simulink model "LED - Simulink scheme"  (R2020b)
settings: Solver=VariableStepAuto  StartTime=0.0  StopTime=10.0  MaxStep=1e-6  RelTol=1e-9
libraries: nesl_utility x28, fl_lib x22, ee_lib x20, simulink x4
settings Model: Creator=claudio.rossi  LastModifiedBy=Gioele
settings SolverCC: ZeroCrossAlgorithm=Adaptive
settings DebuggingCC: IgnoredZcDiagnostic=none
settings SFSimCC: CustomCodeUndefinedFunction=UseInterfaceOnly

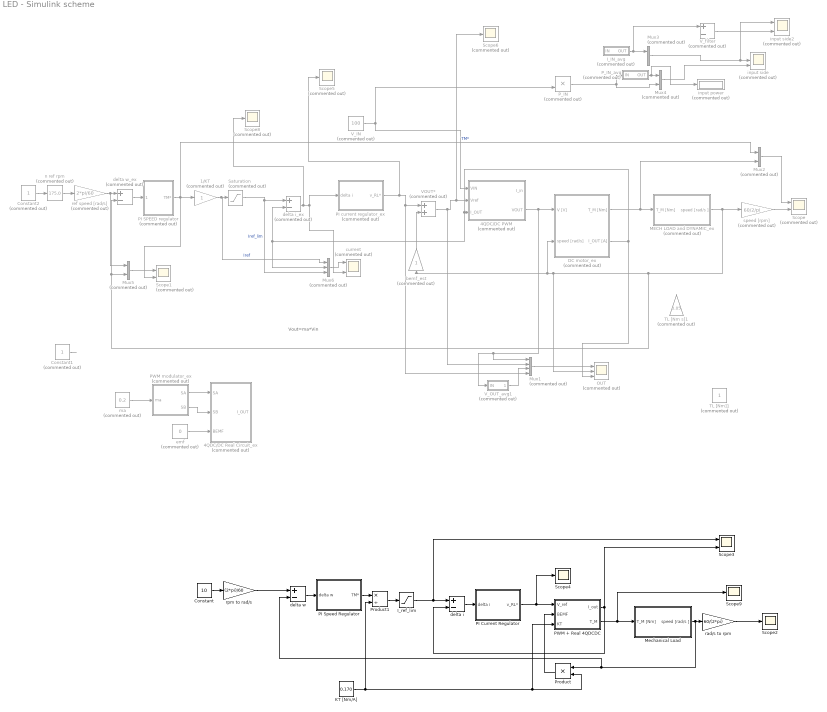
== system LED - Simulink scheme ==
  note: Vout=ma*Vin
  1/KT : Gain  Commented=on
  4QDC/DC PWM : Subsystem  Commented=on
  4QDC/DC Real Circuit_ex : Subsystem  Commented=on
  Constant : Constant  Value=10
  Constant1 : Constant  Commented=on
  Constant2 : Constant  Commented=on
  DC motor_ex : Subsystem  Commented=on
  I_IN_avg : Subsystem  Commented=on  mask{Ts=0.001}
      mask prompts: Ts "period [s]"
  I_ref_lim : Saturate  UpperLimit=1.8  LowerLimit=-1.7
  KT [Nm/A] : Constant  Value=0.170
  MECH LOAD and DYNAMIC_ex : Subsystem  Commented=on
  Mechanical Load : Subsystem
  Mux1 : Mux  Commented=on
  Mux{2..5} (4 alike) : Mux  Commented=on  Inputs=2
  Mux6 : Mux  Commented=on  Inputs=3
  OUT : Scope  Commented=on  NumInputPorts=3
  PI Current Regulator : Subsystem
  PI SPEED regulator : Subsystem  Commented=on
  PI Speed Regulator : Subsystem
  PI current regulator_ex : Subsystem  Commented=on
  "PWM + Real 4QDCDC " : Subsystem
  PWM modulator_ex : Subsystem  Commented=on
  P_IN : Product  Commented=on
  P_IN_avg : Subsystem  Commented=on  mask{Ts=0.001}
      mask prompts: Ts "period [s]"
  Product : Product
  Product1 : Product  Inputs=*/
  Saturation : Saturate  Commented=on  UpperLimit=5  LowerLimit=-5
  Scope : Scope  Commented=on  NumInputPorts=2
  Scope1 : Scope  Commented=on  NumInputPorts=2
  Scope2 : Scope
  Scope3 : Scope  NumInputPorts=2
  Scope4 : Scope
  Scope5 : Scope  Commented=on
  Scope6 : Scope  Commented=on
  Scope8 : Scope  Commented=on
  Scope9 : Scope
  TL [Nm s]1 : Gain  Commented=on  Gain=0.05
  TL [Nm]1 : Constant  Commented=on
  VOUT* : Sum  Commented=on
  V_IN : Constant  Commented=on  Value=100
  V_OUT_avg1 : Subsystem  Commented=on  mask{Ts=0.00005}
      mask prompts: Ts "period"
  V_filter : Sum  Commented=on  Inputs=+-
  bemf_est : Gain  Commented=on
  current : Scope  Commented=on  NumInputPorts=2
  delta i : Sum  Inputs=+-
  delta i_ex : Sum  Commented=on  Inputs=+-
  delta w : Sum  Inputs=+-
  delta w_ex : Sum  Commented=on  Inputs=+-
  emf : Constant  Commented=on  Value=0
  input power : Display  Commented=on
  input side : Scope  Commented=on  NumInputPorts=3
  input side2 : Scope  Commented=on  NumInputPorts=2
  ma : Constant  Commented=on  Value=0.2
  n ref rpm : simulink/Math Operations/Slider Gain  Commented=on  gain=175.0  low=-500  high=1000
  rad/s to rpm : Gain  Gain=60/(2*pi)
  ref speed [rad/s] : Gain  Commented=on  Gain=2*pi/60
  rpm to rad/s : Gain  Gain=(2*pi)/60
  speed [rpm] : Gain  Commented=on  Gain=60/2/pi
  wires:
  ma/1 -> PWM modulator_ex/1(ma)
  PWM modulator_ex/1(SA) -> 4QDC/DC Real Circuit_ex/1(SA)
  PWM modulator_ex/2(SB) -> 4QDC/DC Real Circuit_ex/2(SB)
  emf/1 -> 4QDC/DC Real Circuit_ex/3(BEMF)
  Constant1/1 -> ?
  Saturation/1 -> Mux6/3, delta i_ex/1  "Iref_lim"
  Mux3/1 -> input side2/1, input side/2
  ref speed [rad/s]/1 -> Mux5/1, delta w_ex/1
  Mux5/1 -> Scope1/1
  Constant2/1 -> n ref rpm/1
  delta w_ex/1 -> PI SPEED regulator/1(delta w)
  n ref rpm/1 -> ref speed [rad/s]/1
  speed [rpm]/1 -> Scope/2
  PI SPEED regulator/1(TM*) -> 1/KT/1, Mux2/1, Scope1/2  "TM*"
  DC motor_ex/1(T_M [Nm]) -> Mux2/2, MECH LOAD and DYNAMIC_ex/1(T_M [Nm])
  Mux4/1 -> input side/3
  V_IN/1 -> 4QDC/DC PWM/1(VIN), P_IN/2
  Mux2/1 -> Scope/1
  MECH LOAD and DYNAMIC_ex/1(speed [rad/s ]) -> Mux5/2, delta w_ex/2, OUT/2, bemf_est/1, DC motor_ex/2(speed [rad/s]), speed [rpm]/1
  I_IN_avg/1(OUT) -> V_filter/1, Mux3/1
  Mux6/1 -> current/1
  4QDC/DC PWM/2(VOUT) -> V_OUT_avg1/1(IN), Mux1/1, DC motor_ex/1(V [V])
  PI current regulator_ex/1(v_RL*) -> Scope5/1, Mux1/4, VOUT*/1
  DC motor_ex/2(I_OUT [A]) -> OUT/3, delta i_ex/2, Mux6/2, 4QDC/DC PWM/3(I_OUT)
  V_OUT_avg1/1(OUT) -> Mux1/3
  delta i_ex/1 -> Scope8/1, PI current regulator_ex/1(delta i), current/2
  1/KT/1 -> Mux6/1, Saturation/1  "Iref"
  VOUT*/1 -> Mux1/2, Scope6/1, 4QDC/DC PWM/2(Vref)
  bemf_est/1 -> VOUT*/2
  P_IN/1 -> Mux4/2, P_IN_avg/1(IN)
  P_IN_avg/1(OUT) -> input power/1, Mux4/1
  Mux1/1 -> OUT/1
  V_filter/1 -> input side2/2
  Product/1 -> "PWM + Real 4QDCDC "/2(BEMF)
  "PWM + Real 4QDCDC "/2(T_M) -> Scope9/1, Mechanical Load/1(T_M [Nm])
  KT [Nm/A]/1 -> Product/2, "PWM + Real 4QDCDC "/3(KT), Product1/2
  PI Current Regulator/1(v_RL*) -> Scope4/1, "PWM + Real 4QDCDC "/1(V_ref)
  delta i/1 -> PI Current Regulator/1(delta i)
  Product1/1 -> I_ref_lim/1
  PI Speed Regulator/1(TM*) -> Product1/1
  delta w/1 -> PI Speed Regulator/1(delta w)
  rad/s to rpm/1 -> Scope2/1
  rpm to rad/s/1 -> delta w/1
  Constant/1 -> rpm to rad/s/1
  I_ref_lim/1 -> delta i/1, Scope3/1
  Mechanical Load/1(speed [rad/s ]) -> delta w/2, Product/1, rad/s to rpm/1
  "PWM + Real 4QDCDC "/1(I_out) -> Scope3/2, delta i/2

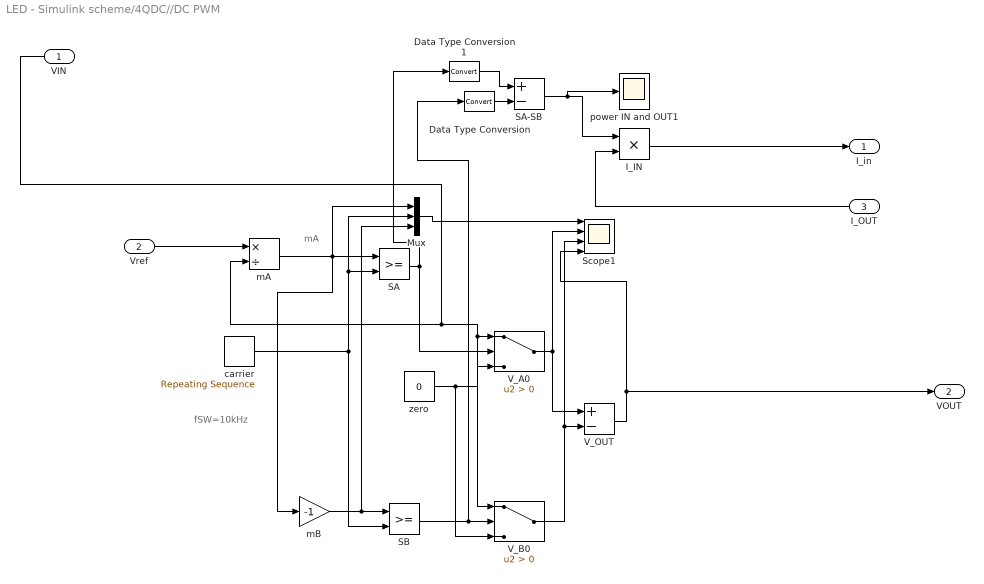
== system LED - Simulink scheme/4QDC//DC PWM ==
  note: mA
  note: fSW=10kHz
  VIN : Inport
  Vref : Inport  Port=2
  I_OUT : Inport  Port=3
  Data Type Conversion : DataTypeConversion
  Data Type Conversion1 : DataTypeConversion
  I_IN : Product
  Mux : Mux  Inputs=3
  SA : RelationalOperator  OutDataTypeStr=boolean  RndMeth=Simplest
  SA-SB : Sum  Inputs=+-
  SB : RelationalOperator  OutDataTypeStr=boolean  RndMeth=Simplest
  Scope1 : Scope  NumInputPorts=4
  V_A0 : Switch  Criteria=u2 > Threshold
  V_B0 : Switch  Criteria=u2 > Threshold
  V_OUT : Sum  Inputs=+-
  carrier : simulink/Sources/Repeating Sequence  rep_seq_t=[0 1e-4/2 1e-4]  rep_seq_y=[-1 1 -1]
  mA : Product  Inputs=*/
  mB : Gain  Gain=-1
  power IN and OUT1 : Scope
  zero : Constant  Value=0
  I_in : Outport  VectorParamsAs1DForOutWhenUnconnected=off
  VOUT : Outport  Port=2  VectorParamsAs1DForOutWhenUnconnected=off
  wires:
  I_IN/1 -> I_in/1
  zero/1 -> V_B0/3, V_A0/3
  carrier/1 -> SB/2, Mux/2, SA/2
  Mux/1 -> Scope1/1
  mA/1 -> mB/1, Mux/1, SA/1
  V_A0/1 -> Scope1/2, V_OUT/1
  VIN/1 -> V_B0/1, V_A0/1, mA/2
  V_OUT/1 -> Scope1/4, VOUT/1
  SA/1 -> Data Type Conversion1/1, V_A0/2
  I_OUT/1 -> I_IN/2
  SB/1 -> Data Type Conversion/1, V_B0/2
  V_B0/1 -> Scope1/3, V_OUT/2
  Data Type Conversion/1 -> SA-SB/2
  SA-SB/1 -> power IN and OUT1/1, I_IN/1
  mB/1 -> SB/1, Mux/3
  Data Type Conversion1/1 -> SA-SB/1
  Vref/1 -> mA/1

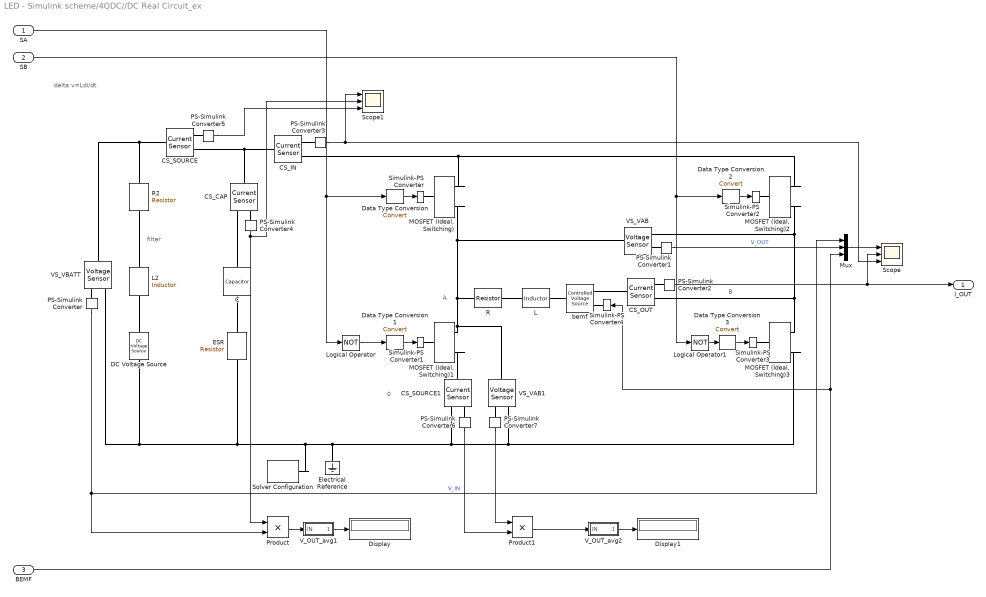
== system LED - Simulink scheme/4QDC//DC Real Circuit_ex ==
  note: filter
  note: B
  note: 0
  note: A
  note: delta v=Ldi/dt
  SA : Inport
  SB : Inport  Port=2
  BEMF : Inport  Port=3
  C : ee_lib/Passive/Capacitor  cap_option=0  c=1e-3 F  Cvec=[1e-05, 1e-06] F  Vvec=[0, 10] V  CV_table_symmetry=1  f_vec=[1, 10] kHz  DFext_vec=[.8, 1.2]  C_tol=5  enable_C_tol=0  tol_distribution=1  nSigma=4  r=1e-6 Ohm  g=0 1/Ohm  averaging_period=0 s  enable_operating_limits=0  operating_limit_action=2  max_working_voltage_range=[-25, 25] V  power_rating=1 W  enable_faults=0  fault_action=1  Cscale_faulted=100  R_faulted=1e-3 Ohm  G_faulted=0 1/Ohm  tau_fault=1e-3 s  enable_temporal_fault=0  t_fault=1 s  enable_behavioral_fault=0  max_permissible_voltage_range=[-100, 100] V  t_fail_on_voltage=1 s  i_specify=off  i_priority=None  i=0 A  i_nominal_specify=off  i_nominal_unit=A  i_nominal_value=1  v_specify=off  v_priority=None  v=0 V  v_nominal_specify=off  v_nominal_unit=V  v_nominal_value=1  vc_specify=off  vc_priority=High  vc=0 V  vc_nominal_specify=off  vc_nominal_unit=V  vc_nominal_value=1
  CS_CAP : fl_lib/Electrical/Electrical Sensors/Current Sensor
  CS_IN : fl_lib/Electrical/Electrical Sensors/Current Sensor
  CS_OUT : fl_lib/Electrical/Electrical Sensors/Current Sensor
  CS_SOURCE : fl_lib/Electrical/Electrical Sensors/Current Sensor
  CS_SOURCE1 : fl_lib/Electrical/Electrical Sensors/Current Sensor
  DC Voltage Source : fl_lib/Electrical/Electrical Sources/DC Voltage Source  v0=100 V
  Data Type Conversion{,1..3} (4 alike) : DataTypeConversion
  Display : Display
  Display1 : Display
  ESR : ee_lib/Passive/Resistor  R=0.01 Ohm  R_tol=5  enable_R_tol=0  tol_distribution=1  nSigma=4  enable_operating_limits=0  operating_limit_action=2  max_working_voltage=100 V  power_rating=1 W  enable_faults=0  fault_action=1  R_faulted=inf Ohm  enable_temporal_fault=0  t_fault=1 s  enable_behavioral_fault=0  max_permissible_current=1 A  t_fail_on_current=1 s  noise_mode=0  sample_time=1e-3 s  repeatability=1  auto_seed=249578223  user_seed=0  Tdevice=25 degC  alpha=3.93e-3 1/K  Tmeas=25 degC  thermal_mass=100 J/K  power_derating_T1=70 degC  power_derating_T2=155 degC  operating_temperature_range_vec=[-50, 150] degC  temperature_specify=off  temperature_priority=High  temperature=298.15 K  temperature_nominal_specify=off  temperature_nominal_unit=K  temperature_nominal_value=1
  Electrical Reference : fl_lib/Electrical/Electrical Elements/Electrical Reference
  L : ee_lib/Passive/Inductor  l=10e-3 H  L_tol=20  enable_L_tol=0  tol_distribution=1  nSigma=4  r=0 Ohm  g=1e-9 1/Ohm  enable_operating_limits=0  operating_limit_action=2  max_working_current=1 A  power_rating=1 W  enable_faults=0  fault_action=1  lambdaPercent=50  k_faulted=0.9999  turnsShort=0  openCct=0  groundShort=0  groundShortG=0 1/Ohm  tau_fault=1e-3 s  enable_temporal_fault=0  t_fault=1 s  enable_behavioral_fault=0  max_permissible_voltage=100 V  n_fail_on_voltage=1  max_permissible_current=1 A  t_fail_on_current=1 s  i_L_specify=off  i_L_priority=High  i_L=0 A  i_L_nominal_specify=off  i_L_nominal_unit=A  i_L_nominal_value=1
  L2 : ee_lib/Passive/Inductor  l=1e-5 H  L_tol=20  enable_L_tol=0  tol_distribution=1  nSigma=4  r=0 Ohm  g=1e-9 1/Ohm  enable_operating_limits=0  operating_limit_action=2  max_working_current=1 A  power_rating=1 W  enable_faults=0  fault_action=1  lambdaPercent=50  k_faulted=0.9999  turnsShort=0  openCct=0  groundShort=0  groundShortG=0 1/Ohm  tau_fault=1e-3 s  enable_temporal_fault=0  t_fault=1 s  enable_behavioral_fault=0  max_permissible_voltage=100 V  n_fail_on_voltage=1  max_permissible_current=1 A  t_fail_on_current=1 s  i_L_specify=off  i_L_priority=High  i_L=0 A  i_L_nominal_specify=off  i_L_nominal_unit=A  i_L_nominal_value=1
  Logical Operator : Logic  Operator=NOT  AllPortsSameDT=off  OutDataTypeStr=boolean
  Logical Operator1 : Logic  Operator=NOT  AllPortsSameDT=off  OutDataTypeStr=boolean
  MOSFET (Ideal, Switching){,1..3} (4 alike) : ee_lib/Semiconductors & Converters/MOSFET (Ideal, Switching)  Rds=0.1 Ohm  Goff=1e-6 1/Ohm  Vth=0.5 V  diode_param=1  diode_Vf=0.8 V  diode_Ron=0.001 Ohm  diode_Goff=1e-5 1/Ohm  diode_C=50e-9 F  diode_iRM=-235 A  diode_iF=300 A  diode_idot=-50 A/us  diode_trr_param=1  diode_trr_factor=3  diode_trr=15 us  diode_Qrr=1500 s*uA  thermal_loss_option=2  Von_data=[0, 1.1, 1.3, 1.45, 1.75, 2.25, 2.7; 0, 1, 1.15, 1.35, 1.7, 2.35, 3] V  Eon_data=[0, .29, 1.43, 2.86, 5.71, 13.14, 22.86; 0, .57, 2.63, 5.14, 10.29, 20.57, 30.29] * 1e-3 J  Eoff_data=[0, .21, 1.07, 2.14, 4.29, 9.86, 17.14; 0, .43, 1.97, 3.86, 7.71, 15.43, 22.71] * 1e-3 J  Tj=[298.15, 398.15] K  Iout_data=[0, 10, 50, 100, 200, 400, 600] A  Eon_scalar=22.86e-3 J  Eoff_scalar=17.14e-3 J  Voff=300 V  Iout_scalar=600 A  diodeModelType=ee.enum.converters.diodeModelType.pwl  diode_IfMat=[.07, .12, .19, 1.75, 4.24, 7.32, 11.2; .16, .3, .72, 2.14, 4.02, 6.35, 9.12] A  diode_TjVec=[25, 125] degC  diode_VfVec=[.5, .7, .9, 1.3, 1.7, 2.1, 2.5] V  thermal_network_parameterization=ee.enum.thermalNetworkTopology.external  Rth=[.03, .2] K/W  Rth_Foster=[.03, .2] K/W  thermal_mass_parameterization=ee.enum.thermalNetwork.timeconstant  thermal_mass=[3, 25] J/K  thermal_mass_Foster=[33, 50] J/K  thermal_time_constant=[.1, 5] s  thermal_time_constant_Foster=[1, 10] s  thermal_mass_initial_temperatures=[25, 25] degC  junction_thermal_mass=0.1 J/K  Tau=1e-4 s  vT_specify=off  vT_priority=None  vT=0 V  vT_nominal_specify=off  vT_nominal_unit=V  vT_nominal_value=1  Qj_specify=off  Qj_priority=None  Qj=0 W  Qj_nominal_specify=off  Qj_nominal_unit=W  Qj_nominal_value=1  junction_temperature_specify=off  junction_temperature_priority=None  junction_temperature=25 degC  junction_temperature_nominal_specify=off  junction_temperature_nominal_unit=degC  junction_temperature_nominal_value=1
  Mux : Mux  Inputs=3
  PS-Simulink Converter{,1..7} (8 alike) : nesl_utility/PS-Simulink Converter  PhysicalDomain=network_engine_domain  SubClassName=ps_output  LeftPortType=input  RightPortType=output  PseudoPeriodic=off  Frequencies=[]  Unit=1  AffineConversion=off
  Product : Product
  Product1 : Product
  R : ee_lib/Passive/Resistor  R=10 Ohm  R_tol=5  enable_R_tol=0  tol_distribution=1  nSigma=4  enable_operating_limits=0  operating_limit_action=2  max_working_voltage=100 V  power_rating=1 W  enable_faults=0  fault_action=1  R_faulted=inf Ohm  enable_temporal_fault=0  t_fault=1 s  enable_behavioral_fault=0  max_permissible_current=1 A  t_fail_on_current=1 s  noise_mode=0  sample_time=1e-3 s  repeatability=1  auto_seed=1734551367  user_seed=0  Tdevice=25 degC  alpha=3.93e-3 1/K  Tmeas=25 degC  thermal_mass=100 J/K  power_derating_T1=70 degC  power_derating_T2=155 degC  operating_temperature_range_vec=[-50, 150] degC  temperature_specify=off  temperature_priority=High  temperature=298.15 K  temperature_nominal_specify=off  temperature_nominal_unit=K  temperature_nominal_value=1
  R2 : ee_lib/Passive/Resistor  R=0.1 Ohm  R_tol=5  enable_R_tol=0  tol_distribution=1  nSigma=4  enable_operating_limits=0  operating_limit_action=2  max_working_voltage=100 V  power_rating=1 W  enable_faults=0  fault_action=1  R_faulted=inf Ohm  enable_temporal_fault=0  t_fault=1 s  enable_behavioral_fault=0  max_permissible_current=1 A  t_fail_on_current=1 s  noise_mode=0  sample_time=1e-3 s  repeatability=1  auto_seed=3714298798  user_seed=0  Tdevice=25 degC  alpha=3.93e-3 1/K  Tmeas=25 degC  thermal_mass=100 J/K  power_derating_T1=70 degC  power_derating_T2=155 degC  operating_temperature_range_vec=[-50, 150] degC  temperature_specify=off  temperature_priority=High  temperature=298.15 K  temperature_nominal_specify=off  temperature_nominal_unit=K  temperature_nominal_value=1
  Scope : Scope  NumInputPorts=3
  Scope1 : Scope  NumInputPorts=3
  Simulink-PS Converter{,1..4} (5 alike) : nesl_utility/Simulink-PS Converter  PhysicalDomain=network_engine_domain  SubClassName=ps_input  LeftPortType=input  RightPortType=output  PseudoPeriodic=off  Frequencies=[]  NoiseDistribution=none  NoiseParameters=[]  Unit=1  AffineConversion=off  FilteringAndDerivatives=provide  SimscapeFilterOrder=1  InputFilterTimeConstant=0.001  UdotUserProvided=0
  Solver Configuration : nesl_utility/Solver Configuration  PhysicalDomain=network_engine_domain  SubClassName=solver  LeftPortType=input  RightPortType=generic  Tones=[]  Harmonics=[]  SimulateNoise=off  Profile=off  UseLocalSampling=off  EnableSwitchedLinearOptims=on  FrequencyDomain=off  UseCCode=off  RelTol=0.001  AbsTol=1e-06  MinStep=1e-09  ToWorkspace=off  RevertToSquareIcSolve=off  NumHomotopyIterations=100  PhasorMode=off  PhasorModeNumHarmonics=1  DoDC=off  ResidualTolerance=1e-09  UseLocalSolver=off  LocalSolverChoice=NE_BACKWARD_EULER_ADVANCER  LocalSolverSampleTime=0.001  DoFixedCost=off  MaxNonlinIter=3  MaxModeIter=2  ComputeImpulses=off  ImpulseIterations=2  LinearAlgebra=auto  EquationFormulation=NE_TIME_EF  DelaysMemoryBudget=1024  AutomaticFiltering=on  FilteringTimeConstant=0.001  PartitionStorageMethod=AS_NEEDED  PartitionMemoryBudget=1024  PartitionMethod=ROBUST
  VS_VAB : fl_lib/Electrical/Electrical Sensors/Voltage Sensor
  VS_VAB1 : fl_lib/Electrical/Electrical Sensors/Voltage Sensor
  VS_VBATT : fl_lib/Electrical/Electrical Sensors/Voltage Sensor
  V_OUT_avg1 : Subsystem  mask{Ts=0.0001}
      mask prompts: Ts "period"
  V_OUT_avg2 : Subsystem  mask{Ts=0.0001}
      mask prompts: Ts "period"
  bemf : fl_lib/Electrical/Electrical Sources/Controlled Voltage Source
  I_OUT : Outport  VectorParamsAs1DForOutWhenUnconnected=off
  wires:
  BEMF/1 -> Simulink-PS Converter4/1, Mux/3
  PS-Simulink Converter2/1 -> Scope/2, I_OUT/1
  PS-Simulink Converter3/1 -> Scope1/1, Scope/3
  Logical Operator/1 -> Data Type Conversion1/1
  SA/1 -> Data Type Conversion/1, Logical Operator/1
  Mux/1 -> Scope/1
  Data Type Conversion/1 -> Simulink-PS Converter/1
  Data Type Conversion1/1 -> Simulink-PS Converter1/1
  PS-Simulink Converter/1 -> Product/2, Mux/1  "V_IN"
  PS-Simulink Converter1/1 -> Mux/2  "V_OUT"
  Data Type Conversion2/1 -> Simulink-PS Converter2/1
  PS-Simulink Converter4/1 -> Product/1, Scope1/2
  PS-Simulink Converter5/1 -> Scope1/3
  Product/1 -> V_OUT_avg1/1(IN)
  V_OUT_avg1/1(OUT) -> Display/1
  PS-Simulink Converter7/1 -> Product1/1
  PS-Simulink Converter6/1 -> Product1/2
  Product1/1 -> V_OUT_avg2/1(IN)
  V_OUT_avg2/1(OUT) -> Display1/1
  Data Type Conversion3/1 -> Simulink-PS Converter3/1
  SB/1 -> Logical Operator1/1, Data Type Conversion2/1
  Logical Operator1/1 -> Data Type Conversion3/1
  connections:
  Simulink-PS Converter1/RConn1 -- "MOSFET (Ideal, Switching)1"/LConn1
  "MOSFET (Ideal, Switching)3"/RConn2 -- DC Voltage Source/RConn1 -- VS_VBATT/RConn2 -- ESR/RConn1 -- Solver Configuration/RConn1 -- Electrical Reference/LConn1 -- CS_SOURCE1/RConn2 -- VS_VAB1/RConn2
  CS_IN/LConn1 -- CS_CAP/LConn1 -- CS_SOURCE/RConn2
  CS_IN/RConn1 -- PS-Simulink Converter3/LConn1
  CS_OUT/RConn1 -- PS-Simulink Converter2/LConn1
  bemf/LConn1 -- L/RConn1
  VS_VBATT/RConn1 -- PS-Simulink Converter/LConn1
  "MOSFET (Ideal, Switching)2"/LConn1 -- Simulink-PS Converter2/RConn1
  VS_VAB/RConn2 -- CS_OUT/RConn2 -- "MOSFET (Ideal, Switching)3"/RConn1 -- "MOSFET (Ideal, Switching)2"/RConn2
  bemf/RConn2 -- CS_OUT/LConn1
  "MOSFET (Ideal, Switching)2"/RConn1 -- "MOSFET (Ideal, Switching)"/RConn1 -- CS_IN/RConn2
  L/LConn1 -- R/RConn1
  Simulink-PS Converter4/RConn1 -- bemf/RConn1
  Simulink-PS Converter/RConn1 -- "MOSFET (Ideal, Switching)"/LConn1
  PS-Simulink Converter1/LConn1 -- VS_VAB/RConn1
  DC Voltage Source/LConn1 -- L2/RConn1
  L2/LConn1 -- R2/RConn1
  C/RConn1 -- ESR/LConn1
  CS_CAP/RConn2 -- C/LConn1
  R2/LConn1 -- VS_VBATT/LConn1 -- CS_SOURCE/LConn1
  CS_CAP/RConn1 -- PS-Simulink Converter4/LConn1
  PS-Simulink Converter5/LConn1 -- CS_SOURCE/RConn1
  CS_SOURCE1/RConn1 -- PS-Simulink Converter6/LConn1
  VS_VAB1/RConn1 -- PS-Simulink Converter7/LConn1
  Simulink-PS Converter3/RConn1 -- "MOSFET (Ideal, Switching)3"/LConn1
  "MOSFET (Ideal, Switching)1"/RConn2 -- CS_SOURCE1/LConn1
  "MOSFET (Ideal, Switching)"/RConn2 -- VS_VAB/LConn1 -- R/LConn1 -- VS_VAB1/LConn1 -- "MOSFET (Ideal, Switching)1"/RConn1

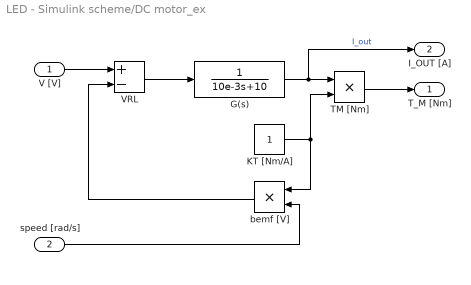
== system LED - Simulink scheme/DC motor_ex ==
  V [V] : Inport
  speed [rad/s] : Inport  Port=2
  G(s) : TransferFcn  Denominator=[10e-3 10]
  KT [Nm/A] : Constant
  TM [Nm] : Product
  VRL : Sum  Inputs=+-
  bemf [V] : Product
  T_M [Nm] : Outport  VectorParamsAs1DForOutWhenUnconnected=off
  I_OUT [A] : Outport  Port=2  VectorParamsAs1DForOutWhenUnconnected=off
  wires:
  TM [Nm]/1 -> T_M [Nm]/1
  V [V]/1 -> VRL/1
  VRL/1 -> G(s)/1
  speed [rad/s]/1 -> bemf [V]/2
  bemf [V]/1 -> VRL/2
  KT [Nm/A]/1 -> TM [Nm]/2, bemf [V]/1
  G(s)/1 -> TM [Nm]/1, I_OUT [A]/1  "I_out"

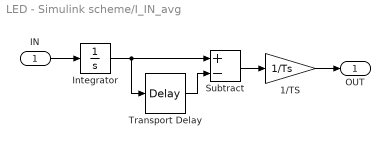
== system LED - Simulink scheme/I_IN_avg ==
  IN : Inport
  1/TS : Gain  Gain=1/Ts
  Integrator : Integrator
  Subtract : Sum  Inputs=+-
  Transport Delay : TransportDelay  DelayTime=Ts
  OUT : Outport  VectorParamsAs1DForOutWhenUnconnected=off
  wires:
  Integrator/1 -> Transport Delay/1, Subtract/1
  1/TS/1 -> OUT/1
  IN/1 -> Integrator/1
  Transport Delay/1 -> Subtract/2
  Subtract/1 -> 1/TS/1

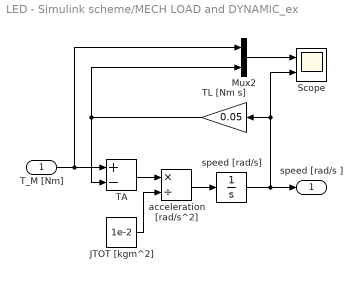
== system LED - Simulink scheme/MECH LOAD and DYNAMIC_ex ==
  T_M [Nm] : Inport
  JTOT [kgm^2] : Constant  Value=1e-2
  Mux2 : Mux  Inputs=2
  Scope : Scope  NumInputPorts=2
  TA : Sum  Inputs=+-
  TL [Nm s] : Gain  Gain=0.05
  acceleration [rad/s^2] : Product  Inputs=*/
  speed [rad/s] : Integrator
  speed [rad/s ] : Outport  VectorParamsAs1DForOutWhenUnconnected=off
  wires:
  T_M [Nm]/1 -> Mux2/1, TA/1
  JTOT [kgm^2]/1 -> acceleration [rad/s^2]/2
  speed [rad/s]/1 -> Scope/2, TL [Nm s]/1, speed [rad/s ]/1
  TA/1 -> acceleration [rad/s^2]/1
  acceleration [rad/s^2]/1 -> speed [rad/s]/1
  TL [Nm s]/1 -> TA/2, Mux2/2
  Mux2/1 -> Scope/1

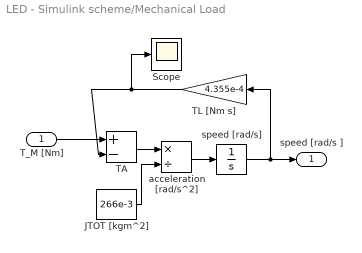
== system LED - Simulink scheme/Mechanical Load ==
  T_M [Nm] : Inport
  JTOT [kgm^2] : Constant  Value=266e-3
  Scope : Scope
  TA : Sum  Inputs=+-
  TL [Nm s] : Gain  Gain=4.355e-4
  acceleration [rad/s^2] : Product  Inputs=*/
  speed [rad/s] : Integrator
  speed [rad/s ] : Outport  VectorParamsAs1DForOutWhenUnconnected=off
  wires:
  TL [Nm s]/1 -> Scope/1, TA/2
  acceleration [rad/s^2]/1 -> speed [rad/s]/1
  TA/1 -> acceleration [rad/s^2]/1
  speed [rad/s]/1 -> speed [rad/s ]/1, TL [Nm s]/1
  JTOT [kgm^2]/1 -> acceleration [rad/s^2]/2
  T_M [Nm]/1 -> TA/1

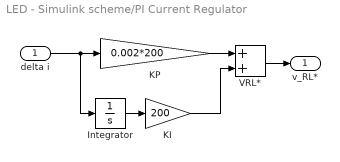
== system LED - Simulink scheme/PI Current Regulator ==
  delta i : Inport
  Integrator : Integrator
  KI : Gain  Gain=200
  KP : Gain  Gain=0.002*200
  VRL* : Sum
  v_RL* : Outport  VectorParamsAs1DForOutWhenUnconnected=off
  wires:
  VRL*/1 -> v_RL*/1
  Integrator/1 -> KI/1
  KI/1 -> VRL*/2
  delta i/1 -> Integrator/1, KP/1
  KP/1 -> VRL*/1

== system LED - Simulink scheme/PI SPEED regulator ==
  delta w : Inport
  Integrator : Integrator
  KI : Gain  Gain=0.08
  KP : Gain  Gain=0.067*0.08
  Tm : Sum
  TM* : Outport  VectorParamsAs1DForOutWhenUnconnected=off
  wires:
  Tm/1 -> TM*/1
  Integrator/1 -> KI/1
  KI/1 -> Tm/2
  delta w/1 -> KP/1, Integrator/1
  KP/1 -> Tm/1

== system LED - Simulink scheme/PI Speed Regulator ==
  delta w : Inport
  Integrator : Integrator
  KI : Gain  Gain=0.08
  KP : Gain  Gain=0.067*0.08
  Tm : Sum
  TM* : Outport  VectorParamsAs1DForOutWhenUnconnected=off
  wires:
  KP/1 -> Tm/1
  Integrator/1 -> KI/1
  delta w/1 -> KP/1, Integrator/1
  Tm/1 -> TM*/1
  KI/1 -> Tm/2

== system LED - Simulink scheme/PI current regulator_ex ==
  delta i : Inport
  Integrator : Integrator
  KI : Gain  Gain=8000
  KP : Gain  Gain=0.00067*8000
  VRL* : Sum
  v_RL* : Outport  VectorParamsAs1DForOutWhenUnconnected=off
  wires:
  KP/1 -> VRL*/1
  delta i/1 -> Integrator/1, KP/1
  KI/1 -> VRL*/2
  Integrator/1 -> KI/1
  VRL*/1 -> v_RL*/1

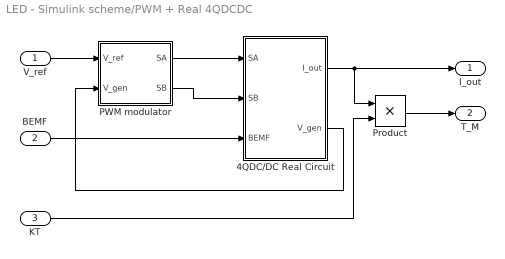
== system LED - Simulink scheme/PWM + Real 4QDCDC  ==
  V_ref : Inport
  BEMF : Inport  Port=2
  KT : Inport  Port=3
  4QDC/DC Real Circuit : Subsystem
  PWM modulator : Subsystem
  Product : Product
  I_out : Outport
  T_M : Outport  Port=2
  wires:
  PWM modulator/1(SA) -> 4QDC/DC Real Circuit/1(SA)
  PWM modulator/2(SB) -> 4QDC/DC Real Circuit/2(SB)
  4QDC/DC Real Circuit/2(V_gen) -> PWM modulator/2(V_gen)
  V_ref/1 -> PWM modulator/1(V_ref)
  BEMF/1 -> 4QDC/DC Real Circuit/3(BEMF)
  4QDC/DC Real Circuit/1(I_out) -> Product/1, I_out/1
  Product/1 -> T_M/1
  KT/1 -> Product/2

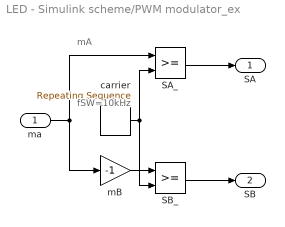
== system LED - Simulink scheme/PWM modulator_ex ==
  note: mA
  note: fSW=10kHz
  ma : Inport
  SA_ : RelationalOperator  OutDataTypeStr=boolean  RndMeth=Simplest
  SB_ : RelationalOperator  OutDataTypeStr=boolean  RndMeth=Simplest
  carrier : simulink/Sources/Repeating Sequence  rep_seq_t=[0 1e-4/2 1e-4]  rep_seq_y=[-1 1 -1]
  mB : Gain  Gain=-1
  SA : Outport  VectorParamsAs1DForOutWhenUnconnected=off
  SB : Outport  Port=2  VectorParamsAs1DForOutWhenUnconnected=off
  wires:
  SA_/1 -> SA/1
  ma/1 -> mB/1, SA_/1
  mB/1 -> SB_/1
  SB_/1 -> SB/1
  carrier/1 -> SA_/2, SB_/2

== system LED - Simulink scheme/P_IN_avg ==
  IN : Inport
  1/TS : Gain  Gain=1/Ts
  Integrator : Integrator
  Subtract : Sum  Inputs=+-
  Transport Delay : TransportDelay  DelayTime=Ts
  OUT : Outport  VectorParamsAs1DForOutWhenUnconnected=off
  wires:
  Integrator/1 -> Transport Delay/1, Subtract/1
  1/TS/1 -> OUT/1
  IN/1 -> Integrator/1
  Transport Delay/1 -> Subtract/2
  Subtract/1 -> 1/TS/1

== system LED - Simulink scheme/V_OUT_avg1 ==
  IN : Inport
  1/TS : Gain  Gain=1/Ts
  Integrator : Integrator
  Subtract : Sum  Inputs=+-
  Transport Delay : TransportDelay  DelayTime=Ts
  OUT : Outport  VectorParamsAs1DForOutWhenUnconnected=off
  wires:
  Subtract/1 -> 1/TS/1
  Transport Delay/1 -> Subtract/2
  IN/1 -> Integrator/1
  1/TS/1 -> OUT/1
  Integrator/1 -> Subtract/1, Transport Delay/1

== system LED - Simulink scheme/4QDC//DC Real Circuit_ex/V_OUT_avg1 ==
  IN : Inport
  1/TS : Gain  Gain=1/Ts
  Integrator : Integrator
  Subtract : Sum  Inputs=+-
  Transport Delay : TransportDelay  DelayTime=Ts
  OUT : Outport  VectorParamsAs1DForOutWhenUnconnected=off
  wires:
  Subtract/1 -> 1/TS/1
  Transport Delay/1 -> Subtract/2
  IN/1 -> Integrator/1
  1/TS/1 -> OUT/1
  Integrator/1 -> Subtract/1, Transport Delay/1

== system LED - Simulink scheme/4QDC//DC Real Circuit_ex/V_OUT_avg2 ==
  IN : Inport
  1/TS : Gain  Gain=1/Ts
  Integrator : Integrator
  Subtract : Sum  Inputs=+-
  Transport Delay : TransportDelay  DelayTime=Ts
  OUT : Outport  VectorParamsAs1DForOutWhenUnconnected=off
  wires:
  Integrator/1 -> Transport Delay/1, Subtract/1
  1/TS/1 -> OUT/1
  IN/1 -> Integrator/1
  Transport Delay/1 -> Subtract/2
  Subtract/1 -> 1/TS/1

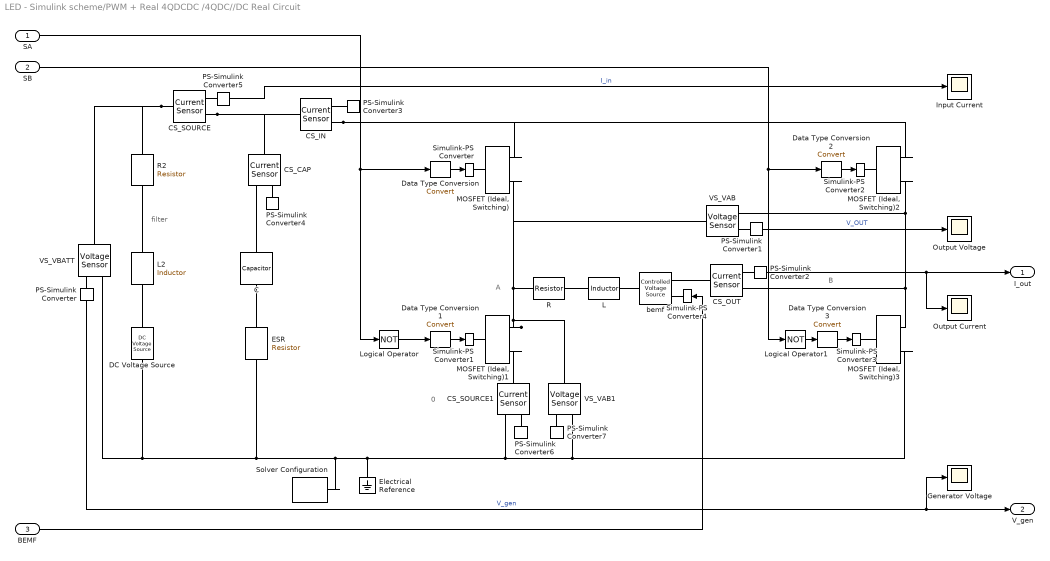
== system LED - Simulink scheme/PWM + Real 4QDCDC /4QDC//DC Real Circuit ==
  note: A
  note: 0
  note: B
  note: filter
  SA : Inport
  SB : Inport  Port=2
  BEMF : Inport  Port=3
  C : ee_lib/Passive/Capacitor  cap_option=0  c=1e-5 F  Cvec=[1e-05, 1e-06] F  Vvec=[0, 10] V  CV_table_symmetry=1  f_vec=[1, 10] kHz  DFext_vec=[.8, 1.2]  C_tol=5  enable_C_tol=0  tol_distribution=1  nSigma=4  r=1e-6 Ohm  g=0 1/Ohm  averaging_period=0 s  enable_operating_limits=0  operating_limit_action=2  max_working_voltage_range=[-25, 25] V  power_rating=1 W  enable_faults=0  fault_action=1  Cscale_faulted=100  R_faulted=1e-3 Ohm  G_faulted=0 1/Ohm  tau_fault=1e-3 s  enable_temporal_fault=0  t_fault=1 s  enable_behavioral_fault=0  max_permissible_voltage_range=[-100, 100] V  t_fail_on_voltage=1 s  i_specify=off  i_priority=None  i=0 A  i_nominal_specify=off  i_nominal_unit=A  i_nominal_value=1  v_specify=off  v_priority=None  v=0 V  v_nominal_specify=off  v_nominal_unit=V  v_nominal_value=1  vc_specify=off  vc_priority=High  vc=0 V  vc_nominal_specify=off  vc_nominal_unit=V  vc_nominal_value=1
  CS_CAP : fl_lib/Electrical/Electrical Sensors/Current Sensor
  CS_IN : fl_lib/Electrical/Electrical Sensors/Current Sensor
  CS_OUT : fl_lib/Electrical/Electrical Sensors/Current Sensor
  CS_SOURCE : fl_lib/Electrical/Electrical Sensors/Current Sensor
  CS_SOURCE1 : fl_lib/Electrical/Electrical Sensors/Current Sensor
  DC Voltage Source : fl_lib/Electrical/Electrical Sources/DC Voltage Source  v0=72 V
  Data Type Conversion{,1..3} (4 alike) : DataTypeConversion
  ESR : ee_lib/Passive/Resistor  R=0.01 Ohm  R_tol=5  enable_R_tol=0  tol_distribution=1  nSigma=4  enable_operating_limits=0  operating_limit_action=2  max_working_voltage=100 V  power_rating=1 W  enable_faults=0  fault_action=1  R_faulted=inf Ohm  enable_temporal_fault=0  t_fault=1 s  enable_behavioral_fault=0  max_permissible_current=1 A  t_fail_on_current=1 s  noise_mode=0  sample_time=1e-3 s  repeatability=1  auto_seed=3499211588  user_seed=0  Tdevice=25 degC  alpha=3.93e-3 1/K  Tmeas=25 degC  thermal_mass=100 J/K  power_derating_T1=70 degC  power_derating_T2=155 degC  operating_temperature_range_vec=[-50, 150] degC  temperature_specify=off  temperature_priority=High  temperature=298.15 K  temperature_nominal_specify=off  temperature_nominal_unit=K  temperature_nominal_value=1
  Electrical Reference : fl_lib/Electrical/Electrical Elements/Electrical Reference
  Generator Voltage : Scope
  Input Current : Scope
  L : ee_lib/Passive/Inductor  l=2.62e-3 H  L_tol=20  enable_L_tol=0  tol_distribution=1  nSigma=4  r=0 Ohm  g=1e-9 1/Ohm  enable_operating_limits=0  operating_limit_action=2  max_working_current=1 A  power_rating=1 W  enable_faults=0  fault_action=1  lambdaPercent=50  k_faulted=0.9999  turnsShort=0  openCct=0  groundShort=0  groundShortG=0 1/Ohm  tau_fault=1e-3 s  enable_temporal_fault=0  t_fault=1 s  enable_behavioral_fault=0  max_permissible_voltage=100 V  n_fail_on_voltage=1  max_permissible_current=1 A  t_fail_on_current=1 s  i_L_specify=off  i_L_priority=High  i_L=0 A  i_L_nominal_specify=off  i_L_nominal_unit=A  i_L_nominal_value=1
  L2 : ee_lib/Passive/Inductor  l=0.72 mH  L_tol=20  enable_L_tol=0  tol_distribution=1  nSigma=4  r=0 Ohm  g=1e-9 1/Ohm  enable_operating_limits=0  operating_limit_action=2  max_working_current=1 A  power_rating=1 W  enable_faults=0  fault_action=1  lambdaPercent=50  k_faulted=0.9999  turnsShort=0  openCct=0  groundShort=0  groundShortG=0 1/Ohm  tau_fault=1e-3 s  enable_temporal_fault=0  t_fault=1 s  enable_behavioral_fault=0  max_permissible_voltage=100 V  n_fail_on_voltage=1  max_permissible_current=1 A  t_fail_on_current=1 s  i_L_specify=off  i_L_priority=High  i_L=0 A  i_L_nominal_specify=off  i_L_nominal_unit=A  i_L_nominal_value=1
  Logical Operator : Logic  Operator=NOT  AllPortsSameDT=off  OutDataTypeStr=boolean
  Logical Operator1 : Logic  Operator=NOT  AllPortsSameDT=off  OutDataTypeStr=boolean
  MOSFET (Ideal, Switching){,1..3} (4 alike) : ee_lib/Semiconductors & Converters/MOSFET (Ideal, Switching)  Rds=0.1 Ohm  Goff=1e-6 1/Ohm  Vth=0.5 V  diode_param=1  diode_Vf=0.8 V  diode_Ron=0.001 Ohm  diode_Goff=1e-5 1/Ohm  diode_C=50e-9 F  diode_iRM=-235 A  diode_iF=300 A  diode_idot=-50 A/us  diode_trr_param=1  diode_trr_factor=3  diode_trr=15 us  diode_Qrr=1500 s*uA  thermal_loss_option=2  Von_data=[0, 1.1, 1.3, 1.45, 1.75, 2.25, 2.7; 0, 1, 1.15, 1.35, 1.7, 2.35, 3] V  Eon_data=[0, .29, 1.43, 2.86, 5.71, 13.14, 22.86; 0, .57, 2.63, 5.14, 10.29, 20.57, 30.29] * 1e-3 J  Eoff_data=[0, .21, 1.07, 2.14, 4.29, 9.86, 17.14; 0, .43, 1.97, 3.86, 7.71, 15.43, 22.71] * 1e-3 J  Tj=[298.15, 398.15] K  Iout_data=[0, 10, 50, 100, 200, 400, 600] A  Eon_scalar=22.86e-3 J  Eoff_scalar=17.14e-3 J  Voff=300 V  Iout_scalar=600 A  diodeModelType=ee.enum.converters.diodeModelType.pwl  diode_IfMat=[.07, .12, .19, 1.75, 4.24, 7.32, 11.2; .16, .3, .72, 2.14, 4.02, 6.35, 9.12] A  diode_TjVec=[25, 125] degC  diode_VfVec=[.5, .7, .9, 1.3, 1.7, 2.1, 2.5] V  thermal_network_parameterization=ee.enum.thermalNetworkTopology.external  Rth=[.03, .2] K/W  Rth_Foster=[.03, .2] K/W  thermal_mass_parameterization=ee.enum.thermalNetwork.timeconstant  thermal_mass=[3, 25] J/K  thermal_mass_Foster=[33, 50] J/K  thermal_time_constant=[.1, 5] s  thermal_time_constant_Foster=[1, 10] s  thermal_mass_initial_temperatures=[25, 25] degC  junction_thermal_mass=0.1 J/K  Tau=1e-4 s  vT_specify=off  vT_priority=None  vT=0 V  vT_nominal_specify=off  vT_nominal_unit=V  vT_nominal_value=1  Qj_specify=off  Qj_priority=None  Qj=0 W  Qj_nominal_specify=off  Qj_nominal_unit=W  Qj_nominal_value=1  junction_temperature_specify=off  junction_temperature_priority=None  junction_temperature=25 degC  junction_temperature_nominal_specify=off  junction_temperature_nominal_unit=degC  junction_temperature_nominal_value=1
  Output Current : Scope
  Output Voltage : Scope
  PS-Simulink Converter{,1..7} (8 alike) : nesl_utility/PS-Simulink Converter  PhysicalDomain=network_engine_domain  SubClassName=ps_output  LeftPortType=input  RightPortType=output  PseudoPeriodic=off  Frequencies=[]  Unit=1  AffineConversion=off
  R : ee_lib/Passive/Resistor  R=10.2 Ohm  R_tol=5  enable_R_tol=0  tol_distribution=1  nSigma=4  enable_operating_limits=0  operating_limit_action=2  max_working_voltage=100 V  power_rating=1 W  enable_faults=0  fault_action=1  R_faulted=inf Ohm  enable_temporal_fault=0  t_fault=1 s  enable_behavioral_fault=0  max_permissible_current=1 A  t_fail_on_current=1 s  noise_mode=0  sample_time=1e-3 s  repeatability=1  auto_seed=3890346746  user_seed=0  Tdevice=25 degC  alpha=3.93e-3 1/K  Tmeas=25 degC  thermal_mass=100 J/K  power_derating_T1=70 degC  power_derating_T2=155 degC  operating_temperature_range_vec=[-50, 150] degC  temperature_specify=off  temperature_priority=High  temperature=298.15 K  temperature_nominal_specify=off  temperature_nominal_unit=K  temperature_nominal_value=1
  R2 : ee_lib/Passive/Resistor  R=0.72 Ohm  R_tol=5  enable_R_tol=0  tol_distribution=1  nSigma=4  enable_operating_limits=0  operating_limit_action=2  max_working_voltage=100 V  power_rating=1 W  enable_faults=0  fault_action=1  R_faulted=inf Ohm  enable_temporal_fault=0  t_fault=1 s  enable_behavioral_fault=0  max_permissible_current=1 A  t_fail_on_current=1 s  noise_mode=0  sample_time=1e-3 s  repeatability=1  auto_seed=545404223  user_seed=0  Tdevice=25 degC  alpha=3.93e-3 1/K  Tmeas=25 degC  thermal_mass=100 J/K  power_derating_T1=70 degC  power_derating_T2=155 degC  operating_temperature_range_vec=[-50, 150] degC  temperature_specify=off  temperature_priority=High  temperature=298.15 K  temperature_nominal_specify=off  temperature_nominal_unit=K  temperature_nominal_value=1
  Simulink-PS Converter{,1..4} (5 alike) : nesl_utility/Simulink-PS Converter  PhysicalDomain=network_engine_domain  SubClassName=ps_input  LeftPortType=input  RightPortType=output  PseudoPeriodic=off  Frequencies=[]  NoiseDistribution=none  NoiseParameters=[]  Unit=1  AffineConversion=off  FilteringAndDerivatives=provide  SimscapeFilterOrder=1  InputFilterTimeConstant=0.001  UdotUserProvided=0
  Solver Configuration : nesl_utility/Solver Configuration  PhysicalDomain=network_engine_domain  SubClassName=solver  LeftPortType=input  RightPortType=generic  Tones=[]  Harmonics=[]  SimulateNoise=off  Profile=off  UseLocalSampling=off  EnableSwitchedLinearOptims=on  FrequencyDomain=off  UseCCode=off  RelTol=0.001  AbsTol=1e-06  MinStep=1e-09  ToWorkspace=off  RevertToSquareIcSolve=off  NumHomotopyIterations=100  PhasorMode=off  PhasorModeNumHarmonics=1  DoDC=off  ResidualTolerance=1e-09  UseLocalSolver=off  LocalSolverChoice=NE_BACKWARD_EULER_ADVANCER  LocalSolverSampleTime=0.001  DoFixedCost=off  MaxNonlinIter=3  MaxModeIter=2  ComputeImpulses=off  ImpulseIterations=2  LinearAlgebra=auto  EquationFormulation=NE_TIME_EF  DelaysMemoryBudget=1024  AutomaticFiltering=on  FilteringTimeConstant=0.001  PartitionStorageMethod=AS_NEEDED  PartitionMemoryBudget=1024  PartitionMethod=ROBUST
  VS_VAB : fl_lib/Electrical/Electrical Sensors/Voltage Sensor
  VS_VAB1 : fl_lib/Electrical/Electrical Sensors/Voltage Sensor
  VS_VBATT : fl_lib/Electrical/Electrical Sensors/Voltage Sensor
  bemf : fl_lib/Electrical/Electrical Sources/Controlled Voltage Source
  I_out : Outport  VectorParamsAs1DForOutWhenUnconnected=off
  V_gen : Outport  Port=2  VectorParamsAs1DForOutWhenUnconnected=off
  wires:
  Logical Operator1/1 -> Data Type Conversion3/1
  SB/1 -> Logical Operator1/1, Data Type Conversion2/1
  Data Type Conversion3/1 -> Simulink-PS Converter3/1
  Data Type Conversion2/1 -> Simulink-PS Converter2/1
  Data Type Conversion1/1 -> Simulink-PS Converter1/1
  Data Type Conversion/1 -> Simulink-PS Converter/1
  SA/1 -> Logical Operator/1, Data Type Conversion/1
  Logical Operator/1 -> Data Type Conversion1/1
  BEMF/1 -> Simulink-PS Converter4/1
  PS-Simulink Converter1/1 -> Output Voltage/1  "V_OUT"
  PS-Simulink Converter2/1 -> I_out/1, Output Current/1
  PS-Simulink Converter5/1 -> Input Current/1  "I_in"
  PS-Simulink Converter/1 -> V_gen/1, Generator Voltage/1  "V_gen"
  connections:
  "MOSFET (Ideal, Switching)1"/RConn1 -- VS_VAB1/LConn1 -- R/LConn1 -- VS_VAB/LConn1 -- "MOSFET (Ideal, Switching)"/RConn2
  "MOSFET (Ideal, Switching)1"/RConn2 -- CS_SOURCE1/LConn1
  Simulink-PS Converter3/RConn1 -- "MOSFET (Ideal, Switching)3"/LConn1
  VS_VAB1/RConn1 -- PS-Simulink Converter7/LConn1
  CS_SOURCE1/RConn1 -- PS-Simulink Converter6/LConn1
  PS-Simulink Converter5/LConn1 -- CS_SOURCE/RConn1
  CS_CAP/RConn1 -- PS-Simulink Converter4/LConn1
  CS_SOURCE/LConn1 -- VS_VBATT/LConn1 -- R2/LConn1
  CS_CAP/RConn2 -- C/LConn1
  C/RConn1 -- ESR/LConn1
  L2/LConn1 -- R2/RConn1
  DC Voltage Source/LConn1 -- L2/RConn1
  PS-Simulink Converter1/LConn1 -- VS_VAB/RConn1
  Simulink-PS Converter/RConn1 -- "MOSFET (Ideal, Switching)"/LConn1
  Simulink-PS Converter4/RConn1 -- bemf/RConn1
  L/LConn1 -- R/RConn1
  CS_IN/RConn2 -- "MOSFET (Ideal, Switching)"/RConn1 -- "MOSFET (Ideal, Switching)2"/RConn1
  bemf/RConn2 -- CS_OUT/LConn1
  "MOSFET (Ideal, Switching)2"/RConn2 -- "MOSFET (Ideal, Switching)3"/RConn1 -- CS_OUT/RConn2 -- VS_VAB/RConn2
  "MOSFET (Ideal, Switching)2"/LConn1 -- Simulink-PS Converter2/RConn1
  VS_VBATT/RConn1 -- PS-Simulink Converter/LConn1
  bemf/LConn1 -- L/RConn1
  CS_OUT/RConn1 -- PS-Simulink Converter2/LConn1
  CS_IN/RConn1 -- PS-Simulink Converter3/LConn1
  CS_SOURCE/RConn2 -- CS_CAP/LConn1 -- CS_IN/LConn1
  VS_VAB1/RConn2 -- CS_SOURCE1/RConn2 -- Electrical Reference/LConn1 -- Solver Configuration/RConn1 -- ESR/RConn1 -- VS_VBATT/RConn2 -- DC Voltage Source/RConn1 -- "MOSFET (Ideal, Switching)3"/RConn2
  Simulink-PS Converter1/RConn1 -- "MOSFET (Ideal, Switching)1"/LConn1

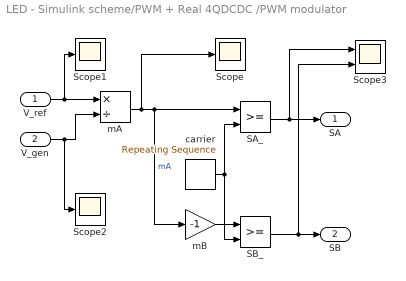
== system LED - Simulink scheme/PWM + Real 4QDCDC /PWM modulator ==
  V_ref : Inport
  V_gen : Inport  Port=2
  SA_ : RelationalOperator  OutDataTypeStr=boolean  RndMeth=Simplest
  SB_ : RelationalOperator  OutDataTypeStr=boolean  RndMeth=Simplest
  Scope : Scope
  Scope1 : Scope
  Scope2 : Scope
  Scope3 : Scope  NumInputPorts=2
  carrier : simulink/Sources/Repeating Sequence  rep_seq_t=[0 5e-5/2 5e-5]  rep_seq_y=[-1 1 -1]
  mA : Product  Inputs=*/
  mB : Gain  Gain=-1
  SA : Outport  VectorParamsAs1DForOutWhenUnconnected=off
  SB : Outport  Port=2  VectorParamsAs1DForOutWhenUnconnected=off
  wires:
  carrier/1 -> SB_/2, SA_/2
  SB_/1 -> Scope3/2, SB/1
  mB/1 -> SB_/1
  mA/1 -> Scope/1, mB/1, SA_/1  "mA"
  SA_/1 -> Scope3/1, SA/1
  V_ref/1 -> Scope1/1, mA/1
  V_gen/1 -> Scope2/1, mA/2
